simulink model "miss04"  (R2024b)
settings: Solver=ode4  StartTime=0.0  StopTime=10.0  FixedStep=2^-7  RelTol=1e-3
libraries: simulink x1
settings Model: Creator=kg53848  LastModifiedBy=kg53848

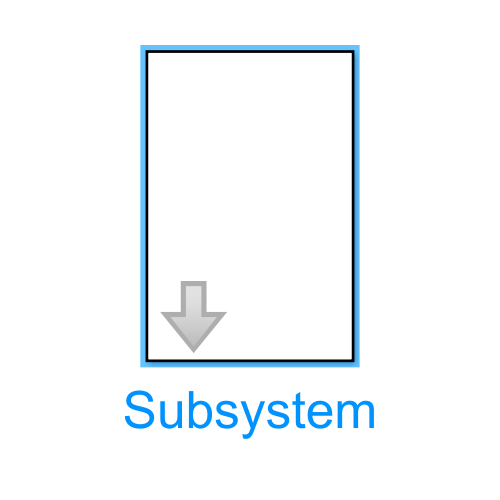
[thumbnail: Simulink's stored preview of the top-level diagram]
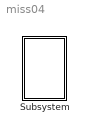
== system miss04 ==
  Subsystem : Subsystem  mask{G=9.81, M=250, rs=0.2, R=3, Vx=10, Vy=5, x=2, y=7}

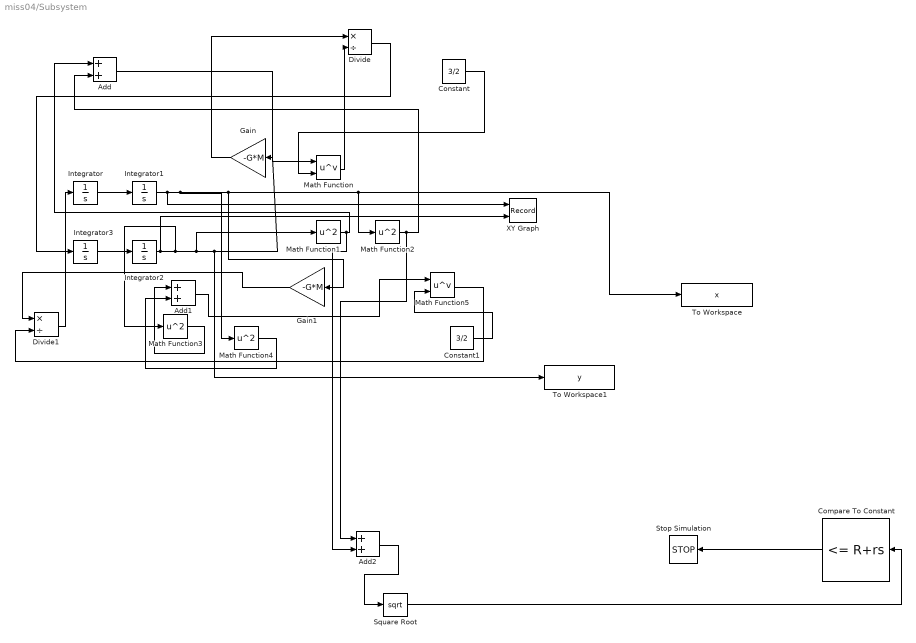
== system miss04/Subsystem ==
  Add : Sum
  Add1 : Sum
  Add2 : Sum
  Compare To Constant : simulink/Logic and Bit Operations/Compare To Constant  relop=<=  const=R+rs  OutDataTypeStr=boolean
  Constant : Constant  Value=3/2
  Constant1 : Constant  Value=3/2
  Divide : Product  Inputs=*/
  Divide1 : Product  Inputs=*/
  Gain : Gain  Gain=-G*M
  Gain1 : Gain  Gain=-G*M
  Integrator : Integrator  InitialCondition=Vx
  Integrator1 : Integrator  InitialCondition=x
  Integrator2 : Integrator  InitialCondition=y
  Integrator3 : Integrator  InitialCondition=Vy
  Math Function : Math  Operator=pow
  Math Function{1..4} (4 alike) : Math  Operator=square
  Math Function5 : Math  Operator=pow
  Square Root : Sqrt
  Stop Simulation : Stop
  To Workspace : ToWorkspace  VariableName=x  SampleTime=-1
  To Workspace1 : ToWorkspace  VariableName=y  SampleTime=-1
  XY Graph : Record  FileSettingsInternal="{\"entries\":[{\"content\":{\"excelSettings\":{\"content\":{},\"type\":\"Streamout.ExcelSettings\"}},\"type\":\"Streamout.FileSettingStorage\",\"uuid\":\"\"}],\"packageUris\":[\"http:\\/\\/schema.mathworks.com\\/mf0\\/streamout_blocks\\/R2020a\"],\"version\":\"1.0\"}"  Layout=[1 1]  SignalsInternal="{\"entries\":[{\"content\":{\"signals\":[{\"content\":{\"blockPath\":[],\"dimensions\":[1],\"domain\":\"\",\"lineColor\":\"#a2142f\",\"plots\":[ 1 ],\"port\":1,\"sid\":[\"\"],\"signalID\":1,\"signalName\":\"Integrator1\"},\"type\":\"RecordBlkView.Signal\",\"uuid\":\"\"},{\"content\":{\"blockPath\":[],\"dimensions\":[1],\"domain\":\"\",\"lineColor\":\"#139fff\",\"plots\":[ 1 ],\"port\":2,\"sid\":[\"\"],\"signalID\":2,\"signalName\":\"Integrator2\"},\"type\":\"RecordBlkView.Signal\",\"uuid\":\"\"}]},\"type\":\"RecordBlkView.InputSignals\",\"uuid\":\"\"}],\"packageUris\":[\"http:\\/\\/schema.mathworks.com\\/mf0\\/streamout_blocks\\/R2020a\"],\"version\":\"1.0\"}"  VisualizationBindings="{\"xyplotplugin\":{\"info\":[{\"series\":[{\"bindingParametersList\":[{\"parameter\":\"X-Axis\",\"signalID\":1,\"signalName\":\"Integrator1\"},{\"parameter\":\"Y-Axis\",\"signalID\":2,\"signalName\":\"Integrator2\"}],\"seriesID\":0}],\"subplotID\":1}]}}"  CompatibilityTag=XY
  wires:
  Math Function4/1 -> Add1/2
  Math Function2/1 -> Add2/1, Add/2
  Add1/1 -> Math Function5/1
  Gain1/1 -> Divide1/1
  Integrator/1 -> Integrator1/1
  Integrator3/1 -> Integrator2/1
  Integrator2/1 -> XY Graph/2, Math Function3/1, Math Function1/1, To Workspace1/1, Gain/1
  Math Function1/1 -> Add2/2, Add/1
  Integrator1/1 -> XY Graph/1, Math Function4/1, To Workspace/1, Math Function2/1, Gain1/1
  Constant/1 -> Math Function/2
  Constant1/1 -> Math Function5/2
  Math Function3/1 -> Add1/1
  Divide1/1 -> Integrator/1
  Math Function/1 -> Divide/2
  Divide/1 -> Integrator3/1
  Add/1 -> Math Function/1
  Gain/1 -> Divide/1
  Math Function5/1 -> Divide1/2
  Compare To Constant/1 -> Stop Simulation/1
  Add2/1 -> Square Root/1
  Square Root/1 -> Compare To Constant/1
